simulink subsystem "PvtSubSys_LONC"  (R2020b)
settings: Solver=VariableStepAuto  StartTime=0.0  StopTime=10.0  RelTol=1e-3
undefined symbols (not defined in the file): P_Global_TireRadius_m, P_Global_Weight_N, P_LongCtrl_VLC_fRollCoef, P_LongCtrl_VLC_WindArea, P_LongCtrl_VLCaccelMinHoldXAxis, P_LongCtrl_VLCaccelMinHoldYAxis, P_LongCtrl_VLCaXCDeadZoneProp_Y, P_LongCtrl_VLCaXCKiCtrlDevChar_Y, P_LongCtrl_VLCaxCtrlDevDeadZoneChar_Y, P_LongCtrl_VLCaxCtrlDevEC2DCMax, P_LongCtrl_VLCaxCtrlDevFastQuitDCMode, P_LongCtrl_VLCaxCtrlDevThresAddEC2DC, P_LongCtrl_VLCaxCtrlDevTresAddDC2EC, P_LongCtrl_VLCAxTarDtThreEnableI, P_LongCtrl_VLCaxvRoadSlopeDC4CharXAxis, P_LongCtrl_VLCaxvRoadSlopeDC4CharYAxis, P_LongCtrl_VLCAxvTracMinDC1FullFillXAxis, P_LongCtrl_VLCAxvTracMinDC1FullFillYAxis, P_LongCtrl_VLCcoefFXAxis, P_LongCtrl_VLCcoefFYAxis, P_LongCtrl_VLCcoefIFadeOut1Calc, P_LongCtrl_VLCcoefIFadeOut1Condition, P_LongCtrl_VLCcoefIFadeOut2Calc, P_LongCtrl_VLCcoefIFadeOut2Condition, P_LongCtrl_VLCcoefIFadeOut3Calc, P_LongCtrl_VLCcoefIFadeOut3Condition, P_LongCtrl_VLCCounterAxvTracMinTimeout, P_LongCtrl_VLCCounterDC2ECTorqDelay, P_LongCtrl_VLCCounterDrvOff2EC, P_LongCtrl_VLCdaxTarEC2DCMax, P_LongCtrl_VLCdriveOffAxUpLimXAxix, P_LongCtrl_VLCdriveOffAxUpLimYAxix, P_LongCtrl_VLCDtAxvRef2UpperBandDC5, P_LongCtrl_VLCIACompensionNeg, P_LongCtrl_VLCIACompensionPos, P_LongCtrl_VLCjerkHoldXAxis, P_LongCtrl_VLCjerkHoldYAxis, P_LongCtrl_VLCki, P_LongCtrl_VLCkp, P_LongCtrl_VLCks, P_LongCtrl_VLCTorqDiffThreAxvTracMinTimeout, P_LongCtrl_VLCTrTatioMax, P_LongCtrl_VLCTrTatioMin, P_LongCtrl_VLCVlcAccThresAxvTracMinTimeout
libraries: simulink x32
(part 2 of 2)

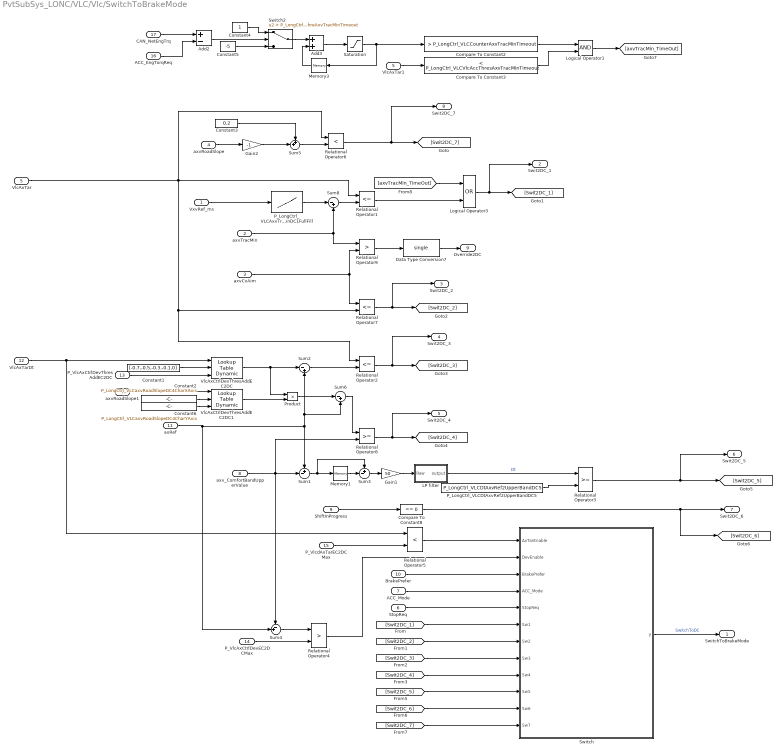
== system PvtSubSys_LONC/VLC/Vlc/SwitchToBrakeMode ==
  VxvRef_ms : Inport
  axvTracMin : Inport  Port=2
  axvCvAim : Inport  Port=3
  axvRoadSlope : Inport  Port=4
  VlcAxTar : Inport  Port=5
  StopReq : Inport  Port=6
  ACC_Mode : Inport  Port=7  OutDataTypeStr=uint8
  axv_ComfortBandUpperValue : Inport  Port=8
  "ShiftInProgress " : Inport  Port=9
  BrakePrefer : Inport  Port=10
  axRef : Inport  Port=11
  VlcAxTarDt : Inport  Port=12
  P_VlcAxCtrlDevThresAddEC2DC : Inport  Port=13
  P_VlcAxCtrlDevEC2DCMax : Inport  Port=14
  P_VlcdAxTarEC2DCMax : Inport  Port=15
  ACC_EngTorqReq : Inport  Port=16  OutDataTypeStr=single
  CAN_NetEngTrq : Inport  Port=17  OutDataTypeStr=single
  Add2 : Sum  Inputs=+-
  Add3 : Sum  AccumDataTypeStr=single
  Compare To Constant2 : simulink/Logic and Bit Operations/Compare To Constant  relop=>  const=P_LongCtrl_VLCCounterAxvTracMinTimeout  OutDataTypeStr=boolean
  Compare To Constant3 : simulink/Logic and Bit Operations/Compare To Constant  relop=<  const=P_LongCtrl_VLCVlcAccThresAxvTracMinTimeout  OutDataTypeStr=boolean
  Compare To Constant8 : simulink/Logic and Bit Operations/Compare To Constant  relop===  const=0  OutDataTypeStr=boolean
  Constant1 : Constant  Value=[-0.7,-0.5,-0.3,-0.1,0]  OutDataTypeStr=single
  Constant2 : Constant  Value=P_LongCtrl_VLCaxvRoadSlopeDC4CharXAxis  OutDataTypeStr=single
  Constant3 : Constant  Value=0.2  OutDataTypeStr=single
  Constant4 : Constant  OutDataTypeStr=single
  Constant5 : Constant  Value=-5  OutDataTypeStr=single
  Constant6 : Constant  Value=P_LongCtrl_VLCaxvRoadSlopeDC4CharYAxis  OutDataTypeStr=single
  Data Type Conversion7 : DataTypeConversion  OutDataTypeStr=single
  Gain1 : Gain  Gain=50
  Gain2 : Gain  Gain=-1
  LP filter : Subsystem
  Logical Operator1 : Logic  AllPortsSameDT=off  OutDataTypeStr=boolean
  Logical Operator3 : Logic  Operator=OR  AllPortsSameDT=off  OutDataTypeStr=boolean
  Memory1 : Memory  InheritSampleTime=on
  Memory3 : Memory  InheritSampleTime=on
  P_LongCtrl_VLCAxvTracMinDC1FullFill : Lookup_n-D  NumberOfTableDimensions=1  BreakpointsForDimension1=P_LongCtrl_VLCAxvTracMinDC1FullFillXAxis  Table=P_LongCtrl_VLCAxvTracMinDC1FullFillYAxis  RndMeth=Simplest  InputSameDT=on
  P_LongCtrl_VLCDtAxvRef2UpperBandDC5 : Constant  Value=P_LongCtrl_VLCDtAxvRef2UpperBandDC5  OutDataTypeStr=single
  Product : Product
  Relational Operator1 : RelationalOperator  Operator=<=  OutDataTypeStr=boolean  RndMeth=Nearest
  Relational Operator2 : RelationalOperator  Operator=<=  OutDataTypeStr=boolean  RndMeth=Nearest
  Relational Operator3 : RelationalOperator  OutDataTypeStr=boolean  RndMeth=Nearest
  Relational Operator4 : RelationalOperator  Operator=>  OutDataTypeStr=boolean  RndMeth=Nearest
  Relational Operator5 : RelationalOperator  Operator=<  OutDataTypeStr=boolean  RndMeth=Nearest
  Relational Operator6 : RelationalOperator  Operator=<  OutDataTypeStr=boolean  RndMeth=Nearest
  Relational Operator7 : RelationalOperator  Operator=<=  OutDataTypeStr=boolean  RndMeth=Nearest
  Relational Operator8 : RelationalOperator  OutDataTypeStr=boolean  RndMeth=Nearest
  Relational Operator9 : RelationalOperator  Operator=>  OutDataTypeStr=boolean  RndMeth=Nearest
  Saturation : Saturate  UpperLimit=100  LowerLimit=0  OutDataTypeStr=single
  Sum1 : Sum  Inputs=+-|
  Sum2 : Sum  Inputs=|-+
  Sum3 : Sum  Inputs=+-|
  Sum4 : Sum  Inputs=-+|
  Sum5 : Sum  Inputs=++|
  Sum6 : Sum  Inputs=|-+
  Sum8 : Sum  Inputs=|-+
  Switch : MATLAB Function  TreatAsAtomicUnit=on
  Switch2 : Switch  Criteria=u2 > Threshold  Threshold=P_LongCtrl_VLCTorqDiffThreAxvTracMinTimeout
  VlcAxCtrlDevThresAddEC2DC : simulink/Lookup Tables/Lookup Table Dynamic  LookUpMeth=Interpolation-Use End Values  OutDataType=fixdt('single')  OutScaling=[]  OutputDataTypeScalingMode=Specify via dialog  OutDataTypeStr=single  DoSatur=off
  VlcAxCtrlDevThresAddEC2DC1 : simulink/Lookup Tables/Lookup Table Dynamic  LookUpMeth=Interpolation-Use End Values  OutDataType=fixdt('single')  OutScaling=[]  OutputDataTypeScalingMode=Specify via dialog  OutDataTypeStr=single  DoSatur=off
  VlcAxTar1 : InportShadow  Port=5
  axvRoadSlope1 : InportShadow  Port=4
  SwitchToBrakeMode : Outport
  Swit2DC_1 : Outport  Port=2
  Swit2DC_2 : Outport  Port=3
  Swit2DC_3 : Outport  Port=4
  Swit2DC_4 : Outport  Port=5
  Swit2DC_5 : Outport  Port=6
  Swit2DC_6 : Outport  Port=7
  Swit2DC_7 : Outport  Port=8
  Override2DC : Outport  Port=9
  wires:
  Product/1 -> Sum6/1
  Constant6/1 -> VlcAxCtrlDevThresAddEC2DC1/3
  axvRoadSlope1/1 -> VlcAxCtrlDevThresAddEC2DC1/1
  VlcAxCtrlDevThresAddEC2DC1/1 -> Product/2
  VlcAxCtrlDevThresAddEC2DC/1 -> Product/1, Sum2/1
  Constant2/1 -> VlcAxCtrlDevThresAddEC2DC1/2
  Sum6/1 -> Relational Operator8/1
  Saturation/1 -> Memory3/1, Compare To Constant2/1
  Relational Operator1/1 -> Logical Operator3/2
  [axvTracMin_TimeOut] -> Logical Operator3/1
  Logical Operator1/1 -> [axvTracMin_TimeOut]
  VlcAxTar1/1 -> Compare To Constant3/1
  ACC_EngTorqReq/1 -> Add2/2
  CAN_NetEngTrq/1 -> Add2/1
  Switch2/1 -> Add3/1
  Constant5/1 -> Switch2/3
  Add2/1 -> Switch2/2
  Compare To Constant3/1 -> Logical Operator1/2
  Compare To Constant2/1 -> Logical Operator1/1
  Add3/1 -> Saturation/1
  Memory3/1 -> Add3/2
  Constant4/1 -> Switch2/1
  Data Type Conversion7/1 -> Override2DC/1
  Relational Operator9/1 -> Data Type Conversion7/1
  axvCvAim/1 -> Relational Operator9/2, Relational Operator7/1
  [Swit2DC_1] -> Switch/6(Sw1)
  [Swit2DC_2] -> Switch/7(Sw2)
  [Swit2DC_3] -> Switch/8(Sw3)
  [Swit2DC_4] -> Switch/9(Sw4)
  [Swit2DC_5] -> Switch/10(Sw5)
  [Swit2DC_6] -> Switch/11(Sw6)
  [Swit2DC_7] -> Switch/12(Sw7)
  StopReq/1 -> Switch/5(StopReq)
  ACC_Mode/1 -> Switch/4(ACC_Mode)
  BrakePrefer/1 -> Switch/3(BrakePrefer)
  Relational Operator4/1 -> Switch/2(DevEnable)
  Relational Operator5/1 -> Switch/1(AxTarEnable)
  Compare To Constant8/1 -> Swit2DC_6/1, [Swit2DC_6]
  "ShiftInProgress "/1 -> Compare To Constant8/1
  Relational Operator3/1 -> Swit2DC_5/1, [Swit2DC_5]
  Relational Operator8/1 -> Swit2DC_4/1, [Swit2DC_4]
  Relational Operator2/1 -> Swit2DC_3/1, [Swit2DC_3]
  Relational Operator7/1 -> [Swit2DC_2], Swit2DC_2/1
  Logical Operator3/1 -> [Swit2DC_1], Swit2DC_1/1
  Relational Operator6/1 -> [Swit2DC_7], Swit2DC_7/1
  Sum5/1 -> Relational Operator6/2
  VlcAxTar/1 -> Relational Operator6/1, Relational Operator1/1, Relational Operator2/1, Relational Operator7/2
  Constant3/1 -> Sum5/1
  Gain2/1 -> Sum5/2
  axvRoadSlope/1 -> Gain2/1
  P_LongCtrl_VLCAxvTracMinDC1FullFill/1 -> Sum8/1
  P_VlcdAxTarEC2DCMax/1 -> Relational Operator5/2
  P_VlcAxCtrlDevEC2DCMax/1 -> Relational Operator4/2
  Sum4/1 -> Relational Operator4/1
  axv_ComfortBandUpperValue/1 -> Sum4/1, Sum1/2, Relational Operator8/2
  P_LongCtrl_VLCDtAxvRef2UpperBandDC5/1 -> Relational Operator3/2
  P_VlcAxCtrlDevThresAddEC2DC/1 -> VlcAxCtrlDevThresAddEC2DC/3
  Constant1/1 -> VlcAxCtrlDevThresAddEC2DC/2
  VlcAxTarDt/1 -> Relational Operator5/1, VlcAxCtrlDevThresAddEC2DC/1
  LP filter/1(output) -> Relational Operator3/1  "Dt"
  Gain1/1 -> LP filter/1(Raw)
  Sum3/1 -> Gain1/1
  Memory1/1 -> Sum3/2
  Sum2/1 -> Relational Operator2/2
  Sum1/1 -> Sum3/1, Memory1/1
  axRef/1 -> Sum1/1, Sum6/2, Sum2/2, Sum4/2
  Switch/1(y) -> SwitchToBrakeMode/1  "SwitchToDC"
  Sum8/1 -> Relational Operator1/2
  axvTracMin/1 -> Sum8/2, Relational Operator9/1
  VxvRef_ms/1 -> P_LongCtrl_VLCAxvTracMinDC1FullFill/1

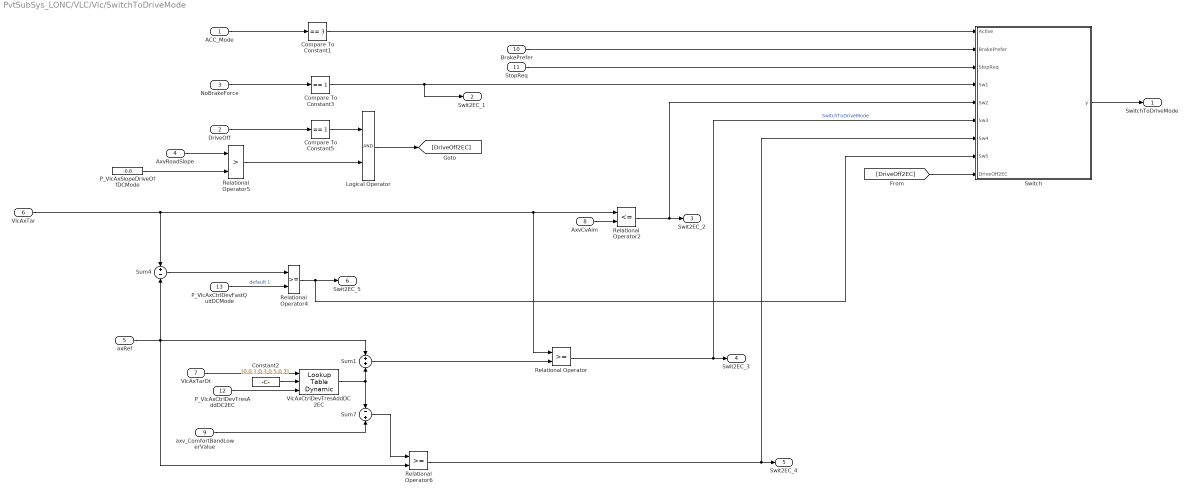
== system PvtSubSys_LONC/VLC/Vlc/SwitchToDriveMode ==
  ACC_Mode : Inport
  DriveOff : Inport  Port=2
  NoBrakeForce : Inport  Port=3
  AxvRoadSlope : Inport  Port=4
  axRef : Inport  Port=5
  VlcAxTar : Inport  Port=6
  VlcAxTarDt : Inport  Port=7
  AxvCvAim : Inport  Port=8
  axv_ComfortBandLowerValue : Inport  Port=9
  BrakePrefer : Inport  Port=10
  StopReq : Inport  Port=11
  P_VlcAxCtrlDevTresAddDC2EC : Inport  Port=12
  P_VlcAxCtrlDevFastQuitDCMode : Inport  Port=13
  Compare To Constant1 : simulink/Logic and Bit Operations/Compare To Constant  relop===  const=3  OutDataTypeStr=boolean
  Compare To Constant3 : simulink/Logic and Bit Operations/Compare To Constant  relop===  const=1  OutDataTypeStr=boolean
  Compare To Constant5 : simulink/Logic and Bit Operations/Compare To Constant  relop===  const=1  OutDataTypeStr=boolean
  Constant2 : Constant  Value=[0,0.1,0.3,0.5,0.7]  OutDataTypeStr=single
  Logical Operator : Logic  AllPortsSameDT=off  OutDataTypeStr=boolean
  P_VlcAxSlopeDriveOffDCMode : Constant  Value=-0.8
  Relational Operator : RelationalOperator  OutDataTypeStr=boolean  RndMeth=Nearest
  Relational Operator2 : RelationalOperator  Operator=<=  OutDataTypeStr=boolean  RndMeth=Nearest
  Relational Operator4 : RelationalOperator  OutDataTypeStr=boolean  RndMeth=Nearest
  Relational Operator5 : RelationalOperator  Operator=>  OutDataTypeStr=boolean  RndMeth=Nearest
  Relational Operator6 : RelationalOperator  OutDataTypeStr=boolean  RndMeth=Nearest
  Sum1 : Sum
  Sum4 : Sum  Inputs=+-
  Sum7 : Sum  Inputs=-+
  Switch : MATLAB Function  TreatAsAtomicUnit=on
  VlcAxCtrlDevTresAddDC2EC : simulink/Lookup Tables/Lookup Table Dynamic  LookUpMeth=Interpolation-Use End Values  OutDataType=fixdt('double')  OutScaling=[]  OutputDataTypeScalingMode=Specify via dialog  OutDataTypeStr=fixdt('double')  DoSatur=off
  SwitchToDriveMode : Outport
  Swit2EC_1 : Outport  Port=2
  Swit2EC_2 : Outport  Port=3
  Swit2EC_3 : Outport  Port=4
  Swit2EC_4 : Outport  Port=5
  Swit2EC_5 : Outport  Port=6
  wires:
  StopReq/1 -> Switch/3(StopReq)
  [DriveOff2EC] -> Switch/9(DriveOff2EC)
  Compare To Constant3/1 -> Switch/4(Sw1), Swit2EC_1/1
  Relational Operator2/1 -> Swit2EC_2/1, Switch/5(Sw2)
  Relational Operator6/1 -> Swit2EC_4/1, Switch/7(Sw4)
  Relational Operator4/1 -> Swit2EC_5/1, Switch/8(Sw5)
  BrakePrefer/1 -> Switch/2(BrakePrefer)
  Sum4/1 -> Relational Operator4/1
  axv_ComfortBandLowerValue/1 -> Sum7/2
  Relational Operator/1 -> Swit2EC_3/1, Switch/6(Sw3)  "SwitchToDriveMode"
  Sum7/1 -> Relational Operator6/1
  Sum1/1 -> Relational Operator/2
  AxvCvAim/1 -> Relational Operator2/2
  VlcAxTar/1 -> Sum4/1, Relational Operator2/1, Relational Operator/1
  Relational Operator5/1 -> Logical Operator/2
  P_VlcAxSlopeDriveOffDCMode/1 -> Relational Operator5/2
  AxvRoadSlope/1 -> Relational Operator5/1
  Switch/1(y) -> SwitchToDriveMode/1
  P_VlcAxCtrlDevFastQuitDCMode/1 -> Relational Operator4/2  "default 1"
  axRef/1 -> Relational Operator6/2, Sum1/1, Sum4/2
  Compare To Constant1/1 -> Switch/1(Active)
  Logical Operator/1 -> [DriveOff2EC]
  Compare To Constant5/1 -> Logical Operator/1
  DriveOff/1 -> Compare To Constant5/1
  ACC_Mode/1 -> Compare To Constant1/1
  VlcAxCtrlDevTresAddDC2EC/1 -> Sum7/1, Sum1/2
  P_VlcAxCtrlDevTresAddDC2EC/1 -> VlcAxCtrlDevTresAddDC2EC/3
  Constant2/1 -> VlcAxCtrlDevTresAddDC2EC/2
  VlcAxTarDt/1 -> VlcAxCtrlDevTresAddDC2EC/1
  NoBrakeForce/1 -> Compare To Constant3/1

== system PvtSubSys_LONC/VLC/Vlc/UpdateFlagCalc ==
  NoBrakeForce : Inport
  DCT_ShiftInProgress : Inport  Port=2
  AxRefDt : Inport  Port=3
  Vxv : Inport  Port=4
  Abs4 : Abs
  Compare To Constant1 : simulink/Logic and Bit Operations/Compare To Constant  relop=<=  const=5  OutDataTypeStr=boolean
  Compare To Constant2 : simulink/Logic and Bit Operations/Compare To Constant  relop=>=  const=18  OutDataTypeStr=boolean
  Compare To Constant4 : simulink/Logic and Bit Operations/Compare To Constant  relop===  const=0  OutDataTypeStr=boolean
  Compare To Constant7 : simulink/Logic and Bit Operations/Compare To Constant  relop===  const=6  OutDataTypeStr=boolean
  Compare To Constant8 : simulink/Logic and Bit Operations/Compare To Constant  relop===  const=0  OutDataTypeStr=boolean
  Logical Operator : Logic  Inputs=5  AllPortsSameDT=off  OutDataTypeStr=boolean
  Sum of Elements1 : Sum  Inputs=+
  Tapped Delay1 : simulink/Discrete/Tapped Delay  vinit=0.0  samptime=-1  NumDelays=5  DelayOrder=Newest  includeCurrent=on
  Timer : Subsystem
  UpdateEnable : Outport
  wires:
  Vxv/1 -> Compare To Constant2/1
  Compare To Constant1/1 -> Logical Operator/2
  Logical Operator/1 -> UpdateEnable/1
  NoBrakeForce/1 -> Tapped Delay1/1
  Timer/1(Timer) -> Compare To Constant4/1
  Compare To Constant7/1 -> Logical Operator/1
  Compare To Constant4/1 -> Logical Operator/5
  DCT_ShiftInProgress/1 -> Compare To Constant8/1, Timer/1(Falling)
  AxRefDt/1 -> Abs4/1
  Tapped Delay1/1 -> Sum of Elements1/1
  Sum of Elements1/1 -> Compare To Constant7/1
  Compare To Constant2/1 -> Logical Operator/3
  Compare To Constant8/1 -> Logical Operator/4
  Abs4/1 -> Compare To Constant1/1

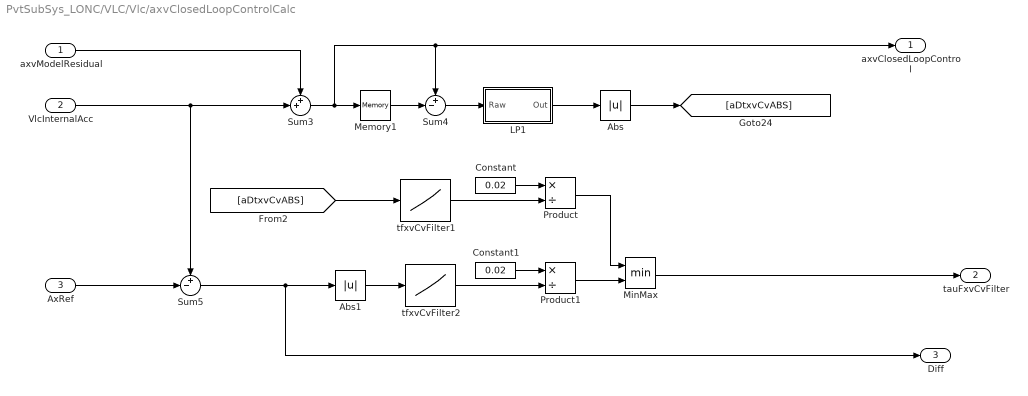
== system PvtSubSys_LONC/VLC/Vlc/axvClosedLoopControlCalc ==
  axvModelResidual : Inport
  VlcInternalAcc : Inport  Port=2
  AxRef : Inport  Port=3
  Abs : Abs
  Abs1 : Abs
  Constant : Constant  Value=0.02  OutDataTypeStr=single
  Constant1 : Constant  Value=0.02  OutDataTypeStr=single
  LP1 : Subsystem
  Memory1 : Memory  InheritSampleTime=on
  MinMax : MinMax  Inputs=2
  Product : Product  Inputs=*/  RndMeth=Zero
  Product1 : Product  Inputs=*/  RndMeth=Zero
  Sum3 : Sum  Inputs=++|
  Sum4 : Sum  Inputs=+-|
  Sum5 : Sum  Inputs=+-|
  "tfxvCvFilter1 " : Lookup_n-D  NumberOfTableDimensions=1  BreakpointsForDimension1=[0,0.1,0.2,1]  Table=[0.1,0.1,0.04,0.04]  RndMeth=Simplest  InputSameDT=on
  tfxvCvFilter2 : Lookup_n-D  NumberOfTableDimensions=1  BreakpointsForDimension1=[0,0.1,0.2,1]  Table=[0.1,0.1,0.02,0.02]  RndMeth=Simplest  InputSameDT=on
  axvClosedLoopControl : Outport
  tauFxvCvFilter : Outport  Port=2
  Diff : Outport  Port=3
  wires:
  AxRef/1 -> Sum5/2
  LP1/1(Out) -> Abs/1
  axvModelResidual/1 -> Sum3/1
  MinMax/1 -> tauFxvCvFilter/1
  Product1/1 -> MinMax/2
  Product/1 -> MinMax/1
  tfxvCvFilter2/1 -> Product1/2
  Constant1/1 -> Product1/1
  "tfxvCvFilter1 "/1 -> Product/2
  Constant/1 -> Product/1
  Abs1/1 -> tfxvCvFilter2/1
  Sum5/1 -> Abs1/1, Diff/1
  VlcInternalAcc/1 -> Sum3/2, Sum5/1
  [aDtxvCvABS] -> "tfxvCvFilter1 "/1
  Abs/1 -> [aDtxvCvABS]
  Sum4/1 -> LP1/1(Raw)
  Memory1/1 -> Sum4/2
  Sum3/1 -> Memory1/1, Sum4/1, axvClosedLoopControl/1

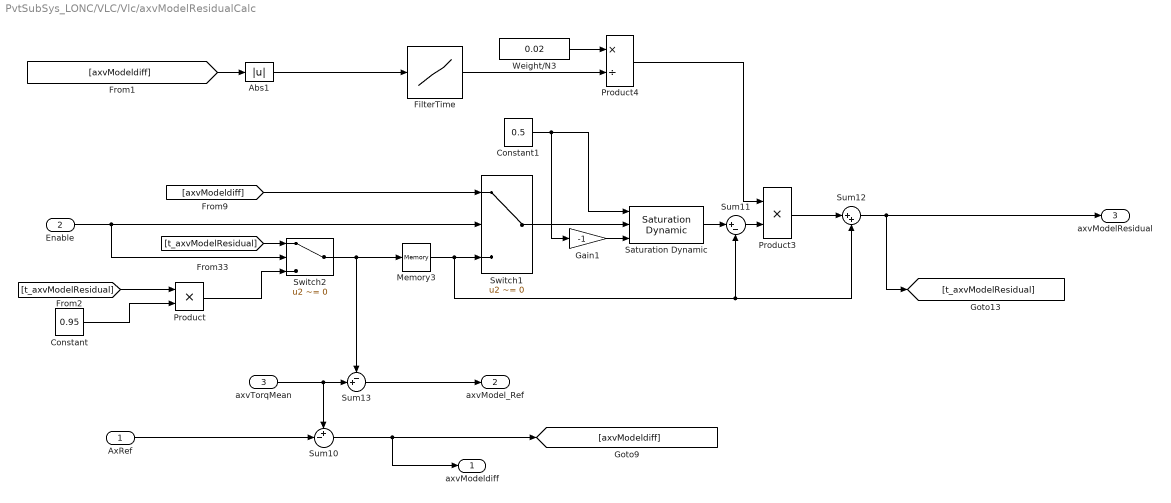
== system PvtSubSys_LONC/VLC/Vlc/axvModelResidualCalc ==
  AxRef : Inport
  Enable : Inport  Port=2
  axvTorqMean : Inport  Port=3
  Abs1 : Abs
  Constant : Constant  Value=0.95  OutDataTypeStr=single
  Constant1 : Constant  Value=0.5  OutDataTypeStr=single
  FilterTime : Lookup_n-D  NumberOfTableDimensions=1  BreakpointsForDimension1=[0,0.1,0.4,0.8,1]  Table=[1,0.4,0.1,0.04,0.04]  RndMeth=Simplest  InputSameDT=on
  Gain1 : Gain  Gain=-1
  Memory3 : Memory  InheritSampleTime=on
  Product : Product  OutDataTypeStr=single
  Product3 : Product  RndMeth=Zero
  Product4 : Product  Inputs=*/  RndMeth=Zero
  Saturation Dynamic : simulink/Discontinuities/Saturation Dynamic  OutMin=[]  OutMax=[]  OutDataTypeStr=Inherit: Same as second input  OutDataType=fixdt(1, 16)  OutScaling=2^-10  DoSatur=off
  Sum10 : Sum  Inputs=+-|
  Sum11 : Sum  Inputs=|+-
  Sum12 : Sum  Inputs=|++
  Sum13 : Sum  Inputs=-+|
  Switch1 : Switch  Criteria=u2 ~= 0
  Switch2 : Switch  Criteria=u2 ~= 0  OutDataTypeStr=single
  Weight/N3 : Constant  Value=0.02  OutDataTypeStr=single  SampleTime=-1
  axvModeldiff : Outport
  axvModel_Ref : Outport  Port=2
  axvModelResidual : Outport  Port=3
  wires:
  Sum13/1 -> axvModel_Ref/1
  Constant/1 -> Product/2
  Constant1/1 -> Saturation Dynamic/1, Gain1/1
  axvTorqMean/1 -> Sum13/2, Sum10/1
  [t_axvModelResidual] -> Switch2/1
  Product3/1 -> Sum12/1
  Saturation Dynamic/1 -> Sum11/1
  [t_axvModelResidual] -> Product/1
  Enable/1 -> Switch1/2, Switch2/2
  Gain1/1 -> Saturation Dynamic/3
  AxRef/1 -> Sum10/2
  [axvModeldiff] -> Abs1/1
  Abs1/1 -> FilterTime/1
  Sum12/1 -> [t_axvModelResidual], axvModelResidual/1
  Sum10/1 -> axvModeldiff/1, [axvModeldiff]
  FilterTime/1 -> Product4/2
  [axvModeldiff] -> Switch1/1
  Switch2/1 -> Memory3/1, Sum13/1
  Product/1 -> Switch2/3
  Memory3/1 -> Switch1/3, Sum11/2, Sum12/2
  Product4/1 -> Product3/1
  Switch1/1 -> Saturation Dynamic/2
  Weight/N3/1 -> Product4/1
  Sum11/1 -> Product3/2

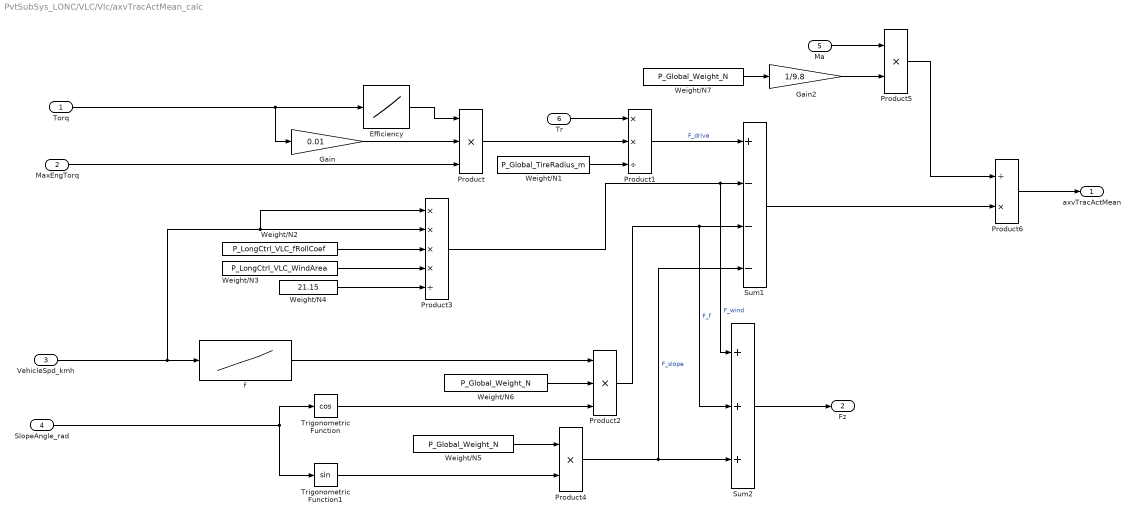
== system PvtSubSys_LONC/VLC/Vlc/axvTracActMean_calc ==
  Torq : Inport  OutDataTypeStr=single
  MaxEngTorq : Inport  Port=2  OutDataTypeStr=single
  VehicleSpd_kmh : Inport  Port=3  OutDataTypeStr=single
  SlopeAngle_rad : Inport  Port=4  OutDataTypeStr=single
  Ma : Inport  Port=5  OutDataTypeStr=single
  Tr : Inport  Port=6  OutDataTypeStr=single
  Efficiency : Lookup_n-D  NumberOfTableDimensions=1  BreakpointsForDimension1=[-100,-20,0,20,100]  Table=[1.10,1.10,1,0.90,0.90]  RndMeth=Simplest  InputSameDT=on
  Gain : Gain  Gain=0.01
  Gain2 : Gain  Gain=1/9.8
  Product : Product  Inputs=***  RndMeth=Zero
  Product1 : Product  Inputs=**/  RndMeth=Zero
  Product2 : Product  Inputs=***  RndMeth=Zero
  Product3 : Product  Inputs=****/  RndMeth=Zero
  Product4 : Product  Inputs=**  RndMeth=Zero
  Product5 : Product  Inputs=**  RndMeth=Zero
  Product6 : Product  Inputs=/*  RndMeth=Zero
  Sum1 : Sum  Inputs=+---
  Sum2 : Sum  Inputs=+++
  Trigonometric Function : Trigonometry  Operator=cos
  Trigonometric Function1 : Trigonometry
  Weight/N1 : Constant  Value=P_Global_TireRadius_m  OutDataTypeStr=single
  Weight/N2 : Constant  Value=P_LongCtrl_VLC_fRollCoef  OutDataTypeStr=single
  Weight/N3 : Constant  Value=P_LongCtrl_VLC_WindArea  OutDataTypeStr=single
  Weight/N4 : Constant  Value=21.15  OutDataTypeStr=single
  Weight/N5 : Constant  Value=P_Global_Weight_N  OutDataTypeStr=single
  Weight/N6 : Constant  Value=P_Global_Weight_N  OutDataTypeStr=single
  Weight/N7 : Constant  Value=P_Global_Weight_N  OutDataTypeStr=single
  f : Lookup_n-D  NumberOfTableDimensions=1  BreakpointsForDimension1=P_LongCtrl_VLCcoefFXAxis  Table=P_LongCtrl_VLCcoefFYAxis  RndMeth=Simplest  InputSameDT=on
  axvTracActMean : Outport  OutDataTypeStr=single
  Fz : Outport  Port=2  OutDataTypeStr=single
  wires:
  f/1 -> Product2/1
  Weight/N1/1 -> Product1/3
  Weight/N5/1 -> Product4/1
  Weight/N6/1 -> Product2/2
  Weight/N7/1 -> Gain2/1
  Sum2/1 -> Fz/1
  Trigonometric Function1/1 -> Product4/2
  Product6/1 -> axvTracActMean/1
  MaxEngTorq/1 -> Product/3
  Tr/1 -> Product1/1
  Ma/1 -> Product5/1
  Gain2/1 -> Product5/2
  Product5/1 -> Product6/1
  Sum1/1 -> Product6/2
  Product4/1 -> Sum1/4, Sum2/3  "F_slope"
  Product2/1 -> Sum1/3, Sum2/2  "F_f"
  Product3/1 -> Sum1/2, Sum2/1  "F_wind"
  Weight/N4/1 -> Product3/5
  Weight/N3/1 -> Product3/4
  Weight/N2/1 -> Product3/3
  Product1/1 -> Sum1/1  "F_drive"
  Trigonometric Function/1 -> Product2/3
  SlopeAngle_rad/1 -> Trigonometric Function1/1, Trigonometric Function/1
  VehicleSpd_kmh/1 -> Product3/1, Product3/2, f/1
  Product/1 -> Product1/2
  Gain/1 -> Product/2
  Efficiency/1 -> Product/1
  Torq/1 -> Efficiency/1, Gain/1

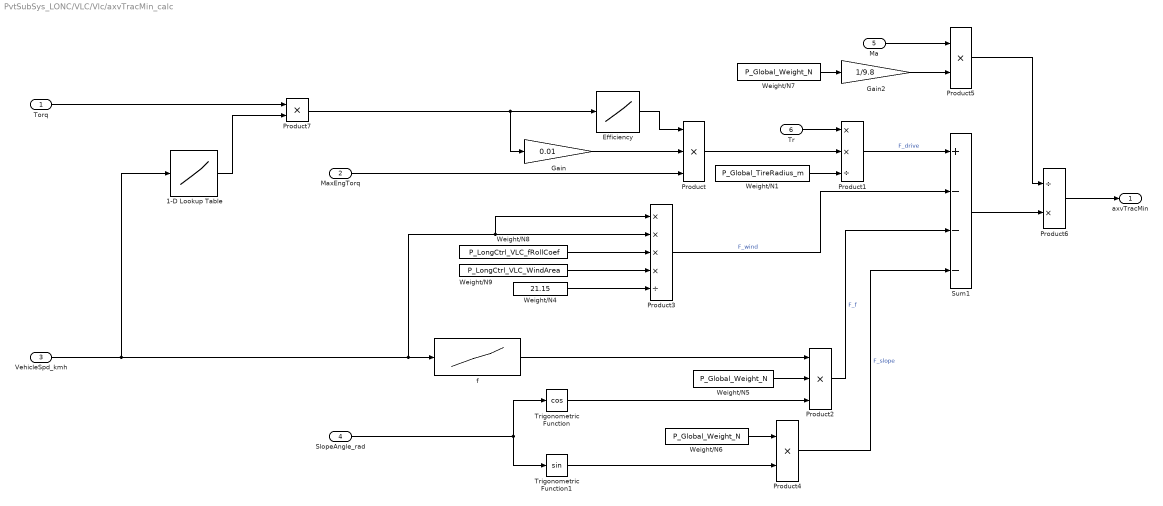
== system PvtSubSys_LONC/VLC/Vlc/axvTracMin_calc ==
  Torq : Inport
  MaxEngTorq : Inport  Port=2
  VehicleSpd_kmh : Inport  Port=3
  SlopeAngle_rad : Inport  Port=4
  Ma : Inport  Port=5
  Tr : Inport  Port=6
  1-D Lookup Table : Lookup_n-D  NumberOfTableDimensions=1  BreakpointsForDimension1=[0 10 20 30 40 50 60 70 80 90 100]  Table=[0 0 0.1 0.65 0.75 0.8 0.85 0.9 0.95 1 1]  ExtrapMethod=Clip  InternalRulePriority=Speed  RndMeth=Simplest  InputSameDT=on
  Efficiency : Lookup_n-D  NumberOfTableDimensions=1  BreakpointsForDimension1=[-100,-20,0,20,100]  Table=[1.10,1.10,1,0.90,0.90]  RndMeth=Simplest  InputSameDT=on
  Gain : Gain  Gain=0.01
  Gain2 : Gain  Gain=1/9.8
  Product : Product  Inputs=***  RndMeth=Zero
  Product1 : Product  Inputs=**/  RndMeth=Zero
  Product2 : Product  Inputs=***  RndMeth=Zero
  Product3 : Product  Inputs=****/  RndMeth=Zero
  Product4 : Product  Inputs=**  RndMeth=Zero
  Product5 : Product  Inputs=**  RndMeth=Zero
  Product6 : Product  Inputs=/*  RndMeth=Zero
  Product7 : Product
  Sum1 : Sum  Inputs=+---
  Trigonometric Function : Trigonometry  Operator=cos
  Trigonometric Function1 : Trigonometry
  Weight/N1 : Constant  Value=P_Global_TireRadius_m  OutDataTypeStr=single
  Weight/N4 : Constant  Value=21.15  OutDataTypeStr=single
  Weight/N5 : Constant  Value=P_Global_Weight_N  OutDataTypeStr=single
  Weight/N6 : Constant  Value=P_Global_Weight_N  OutDataTypeStr=single
  Weight/N7 : Constant  Value=P_Global_Weight_N  OutDataTypeStr=single
  Weight/N8 : Constant  Value=P_LongCtrl_VLC_fRollCoef  OutDataTypeStr=single
  Weight/N9 : Constant  Value=P_LongCtrl_VLC_WindArea  OutDataTypeStr=single
  f : Lookup_n-D  NumberOfTableDimensions=1  BreakpointsForDimension1=P_LongCtrl_VLCcoefFXAxis  Table=P_LongCtrl_VLCcoefFYAxis  RndMeth=Simplest  InputSameDT=on
  axvTracMin : Outport
  wires:
  Torq/1 -> Product7/1
  1-D Lookup Table/1 -> Product7/2
  Product7/1 -> Efficiency/1, Gain/1
  Tr/1 -> Product1/1
  Ma/1 -> Product5/1
  f/1 -> Product2/1
  Weight/N1/1 -> Product1/3
  Weight/N6/1 -> Product4/1
  Weight/N5/1 -> Product2/2
  Weight/N7/1 -> Gain2/1
  Trigonometric Function1/1 -> Product4/2
  Product6/1 -> axvTracMin/1
  MaxEngTorq/1 -> Product/3
  Gain2/1 -> Product5/2
  Product5/1 -> Product6/1
  Sum1/1 -> Product6/2
  Product4/1 -> Sum1/4  "F_slope"
  Product2/1 -> Sum1/3  "F_f"
  Product3/1 -> Sum1/2  "F_wind"
  Weight/N4/1 -> Product3/5
  Weight/N9/1 -> Product3/4
  Weight/N8/1 -> Product3/3
  Product1/1 -> Sum1/1  "F_drive"
  Trigonometric Function/1 -> Product2/3
  SlopeAngle_rad/1 -> Trigonometric Function1/1, Trigonometric Function/1
  VehicleSpd_kmh/1 -> Product3/1, Product3/2, f/1, 1-D Lookup Table/1
  Product/1 -> Product1/2
  Gain/1 -> Product/2
  Efficiency/1 -> Product/1

== system PvtSubSys_LONC/VLC/Vlc/EC/LP ==
  Raw : Inport
  Constant1 : Constant  Value=0.05  OutDataTypeStr=single
  Constant3 : Constant  Value=0.02  OutDataTypeStr=single
  Memory8 : Memory  InheritSampleTime=on
  Product7 : Product  Inputs=*/  RndMeth=Zero
  Product8 : Product  RndMeth=Zero
  Sum14 : Sum
  Sum9 : Sum  Inputs=|+-
  Out : Outport
  wires:
  Constant1/1 -> Product7/2
  Constant3/1 -> Product7/1
  Sum9/1 -> Product8/2
  Sum14/1 -> Memory8/1, Out/1
  Memory8/1 -> Sum14/2, Sum9/2
  Raw/1 -> Sum9/1
  Product8/1 -> Sum14/1
  Product7/1 -> Product8/1

== system PvtSubSys_LONC/VLC/Vlc/FF_Control/L  P ==
  Raw : Inport
  VxvRef : Inport  Port=2
  Constant2 : Constant  Value=0.02  OutDataTypeStr=single
  FilterTime : Lookup_n-D  NumberOfTableDimensions=1  BreakpointsForDimension1=[0,10,20,30,40]  Table=[0.5,0.5,2,3,3]  RndMeth=Simplest  InputSameDT=on
  Memory4 : Memory  InheritSampleTime=on
  Product2 : Product  Inputs=*/  RndMeth=Zero
  Product6 : Product  OutDataTypeStr=single  RndMeth=Zero
  Sum6 : Sum  Inputs=+-
  Sum7 : Sum
  Out : Outport
  wires:
  VxvRef/1 -> FilterTime/1
  Raw/1 -> Sum6/1
  Product6/1 -> Sum7/1
  Product2/1 -> Product6/1
  Sum6/1 -> Product6/2
  FilterTime/1 -> Product2/2
  Constant2/1 -> Product2/1
  Memory4/1 -> Sum7/2, Sum6/2
  Sum7/1 -> Memory4/1, Out/1

== system PvtSubSys_LONC/VLC/Vlc/FF_Control/LP ==
  Raw : Inport
  tauFxvCvFilter : Inport  Port=2
  Add2 : Sum  Inputs=+-
  Add3 : Sum
  Memory : Memory  InheritSampleTime=on
  Product4 : Product  Inputs=**  RndMeth=Zero
  Out : Outport
  wires:
  tauFxvCvFilter/1 -> Product4/1
  Product4/1 -> Add3/1
  Add3/1 -> [FxvCv]
  Add2/1 -> Product4/2
  Memory/1 -> Add2/2, Add3/2
  [FxvCv] -> Memory/1, Out/1
  Raw/1 -> Add2/1

== system PvtSubSys_LONC/VLC/Vlc/PI_Control/If Action Subsystem ==
  In1 : Inport
  Action Port : ActionPort
  Out1 : Outport
  wires:
  In1/1 -> Out1/1

== system PvtSubSys_LONC/VLC/Vlc/PI_Control/If Action Subsystem1 ==
  In1 : Inport
  Action Port : ActionPort
  Gain2 : Gain  Gain=-1
  Out1 : Outport
  wires:
  Gain2/1 -> Out1/1
  In1/1 -> Gain2/1

== system PvtSubSys_LONC/VLC/Vlc/SwitchToBrakeMode/LP filter ==
  Raw : Inport
  FilterTime : Constant  Value=0.1  OutDataTypeStr=single
  Memory2 : Memory  InheritSampleTime=on
  Product1 : Product  RndMeth=Zero
  Product4 : Product  Inputs=*/  RndMeth=Zero
  Sum4 : Sum  Inputs=+-|
  Sum5 : Sum  Inputs=++|
  Weight/N3 : Constant  Value=0.02  OutDataTypeStr=single
  output : Outport
  wires:
  Memory2/1 -> Sum4/2, Sum5/2
  Sum4/1 -> Product1/2
  Sum5/1 -> Memory2/1, output/1
  Product1/1 -> Sum5/1
  Raw/1 -> Sum4/1
  Weight/N3/1 -> Product4/1
  Product4/1 -> Product1/1
  FilterTime/1 -> Product4/2

== system PvtSubSys_LONC/VLC/Vlc/UpdateFlagCalc/Timer ==
  Falling : Inport
  Detect Decrease : simulink/Logic and Bit Operations/Detect Decrease  vinit=0.0  OutDataTypeStr=uint8
  MATLAB Function : MATLAB Function  TreatAsAtomicUnit=on
  Unit Delay : UnitDelay  SampleTime=-1  HasFrameUpgradeWarning=on
  Unit Delay1 : UnitDelay  SampleTime=-1  HasFrameUpgradeWarning=on
  Timer : Outport
  wires:
  Unit Delay/1 -> MATLAB Function/3(StartTimerK1)
  Detect Decrease/1 -> MATLAB Function/1(Falling)
  Unit Delay1/1 -> MATLAB Function/2(TimerK1)
  MATLAB Function/2(StartTimer) -> Unit Delay/1
  Falling/1 -> Detect Decrease/1
  MATLAB Function/1(Timer) -> Unit Delay1/1, Timer/1

== system PvtSubSys_LONC/VLC/Vlc/axvClosedLoopControlCalc/LP1 ==
  Raw : Inport
  Constant3 : Constant  Value=0.02  OutDataTypeStr=single
  FilterTime2 : Constant  Value=0.1  OutDataTypeStr=single
  Memory8 : Memory  InheritSampleTime=on
  Product7 : Product  Inputs=*/  RndMeth=Zero
  Product8 : Product  RndMeth=Zero
  Sum14 : Sum
  Sum9 : Sum  Inputs=+-
  Out : Outport
  wires:
  Constant3/1 -> Product7/1
  FilterTime2/1 -> Product7/2
  Sum9/1 -> Product8/2
  Sum14/1 -> Memory8/1, Out/1
  Memory8/1 -> Sum14/2, Sum9/2
  Raw/1 -> Sum9/1
  Product8/1 -> Sum14/1
  Product7/1 -> Product8/1

== stateflow chart PvtSubSys_LONC/VLC/Vlc/DC/StandstillAccel2 ==
  (default) -> (junction 1)
  (junction 1) -> (junction 3) [order 1] : [ACCmode(1)==6||ACCmode(1)==9]
  (junction 1) -> (junction 7) [order 2] : {timer=single(0);
      | decelReq=VlcAxTar;}
  (junction 3) -> (junction 5) : {timer=min(single(100),timer+single(1));
      |  Ax=min(single(-0.3),VlcAxTar);
      | decelReq=max(accelHoldMin,(Ax+jerkHold*single(0.02)*timer));}
  (junction 5) -> (junction 7)
  (junction 7) -> (junction 14)
  (junction 14) -> (junction 19) [order 1] : [(ACCmode(2)==6||ACCmode(2)==9)&&(ACCmode(1)==7)]
  (junction 14) -> (junction 23) [order 2] : {timerFailure=max(uint8(0),timerFailure-uint8(1));}
  (junction 19) -> (junction 21) : {timerFailure=uint8(75);}
  (junction 21) -> (junction 23)
  (junction 23) -> (junction 26)
  (junction 26) -> (junction 28) [order 1] : [timerFailure>0]
  (junction 26) -> (junction 32) [order 2] : {decelReqActive=false;}
  (junction 28) -> (junction 30) : {decelReq=decelReqK1;
      |  decelReqActive=true;}
  (junction 30) -> (junction 32)
  (junction 32) -> (junction 35) : {decelReqK1=decelReq;}
  data: decelReqActive output; VlcAxTar input single; ACCmode input; timer local single =single(0); decelReq output single; Ax local; accelHoldMin input; jerkHold input single; timerFailure local =uint8(0); decelReqK1 local

== matlab function PvtSubSys_LONC/VLC/Vlc/EC/FxLimit ==
  data: tEC input single; Up output single; UpDelta input single; VxvRef input single; LowDelta input single; DCK1 input boolean; EC input boolean; Driveoff input boolean; CounterK1 input single; Low output single; Counter output single; Counter2K1 input single; Counter2 output single; P_LongCtrl_VLCCounterDrvOff2EC parameter single; P_LongCtrl_VLCCounterDC2ECTorqDelay parameter single
function [Up,Low,Counter,Counter2] = fcn(tEC,UpDelta,VxvRef,LowDelta,DCK1,EC,Driveoff,CounterK1,Counter2K1, P_LongCtrl_VLCCounterDrvOff2EC, P_LongCtrl_VLCCounterDC2ECTorqDelay)
%#codegen
Counter = single(max(CounterK1-1,single(0))); 
Counter2 = single(max(Counter2K1-1,single(0))); 
if ((Driveoff(1)==1)&&(Driveoff(2)==0))
    Counter=P_LongCtrl_VLCCounterDrvOff2EC;             
else
    if (VxvRef>0.3)&&(EC(1)==1)&&(DCK1==1)
        Counter2=P_LongCtrl_VLCCounterDC2ECTorqDelay;         
    end
end
if ( Counter>0)
    Up=single(0);
    Low=single(0);
else
    Up = min(tEC*single(0.5),UpDelta);
    Low = max(-tEC, LowDelta);
    if Counter2>0
        Up = min(tEC*single(0.1),UpDelta);
    end
end

== matlab function PvtSubSys_LONC/VLC/Vlc/EC/MATLAB Function ==
  data: EngTorq_k1 input; NetEngTorq input; y output; EC_enable_k1 input
function y = fcn(EngTorq_k1,NetEngTorq,EC_enable_k1)
%#codegen
if EC_enable_k1==0
    y = NetEngTorq;
else
    y = EngTorq_k1;
end

== matlab function PvtSubSys_LONC/VLC/Vlc/PI_Control/MATLAB Function ==
  data: I_k1 input single; Err input single; ECenable input boolean; I output single; Limited output single; axvFilt output single; Diff input single; tCycle input single; P_VlcWindupLim input single; AxTarDt input single; axv input single; tConst input single; VlcAxTar input single; ShiftInProgress input boolean; axvFiltK1 input single; P_LongCtrl_VLCAxTarDtThreEnableI parameter single; P_LongCtrl_VLCcoefIFadeOut1Condition parameter single; P_LongCtrl_VLCcoefIFadeOut1Calc parameter single; P_LongCtrl_VLCcoefIFadeOut2Condition parameter single; P_LongCtrl_VLCcoefIFadeOut2Calc parameter single; P_LongCtrl_VLCcoefIFadeOut3Condition parameter single; P_LongCtrl_VLCcoefIFadeOut3Calc parameter single; P_LongCtrl_VLCIACompensionPos parameter single; P_LongCtrl_VLCIACompensionNeg parameter single
function [I,Limited,axvFilt] = calcI(I_k1,Err,ECenable,Diff,tCycle,P_VlcWindupLim,AxTarDt,axv,tConst,VlcAxTar,ShiftInProgress,axvFiltK1,P_LongCtrl_VLCAxTarDtThreEnableI, P_LongCtrl_VLCcoefIFadeOut1Condition, P_LongCtrl_VLCcoefIFadeOut1Calc, P_LongCtrl_VLCcoefIFadeOut2Condition, P_LongCtrl_VLCcoefIFadeOut2Calc,...
      P_LongCtrl_VLCcoefIFadeOut3Condition, P_LongCtrl_VLCcoefIFadeOut3Calc, P_LongCtrl_VLCIACompensionPos, P_LongCtrl_VLCIACompensionNeg)
tau=tCycle/tConst;
axvFilt=tau*(axv-axvFiltK1)+axvFiltK1;
if ShiftInProgress==0
    if (((I_k1>0)&&(Diff>0))||((I_k1<=0)&&(Diff<=0)))&&(abs(AxTarDt)<P_LongCtrl_VLCAxTarDtThreEnableI)
         t_I =Diff*tCycle;   
    else
         if abs(Diff)>P_LongCtrl_VLCcoefIFadeOut1Condition*Err
             t_I =P_LongCtrl_VLCcoefIFadeOut1Calc*Diff*tCycle;
         elseif abs(Diff)>P_LongCtrl_VLCcoefIFadeOut2Condition*Err
                 t_I =P_LongCtrl_VLCcoefIFadeOut2Calc*Diff*tCycle;
             elseif abs(Diff)>P_LongCtrl_VLCcoefIFadeOut3Condition*Err
                     t_I =P_LongCtrl_VLCcoefIFadeOut3Calc*Diff*tCycle;
                 else 
                     t_I =Diff*tCycle;
         end       
    end
    if ((abs(AxTarDt)<P_LongCtrl_VLCAxTarDtThreEnableI)&&(abs(Diff)<Err))
         if (abs(VlcAxTar)>0.001&&(abs(axvFilt)<Err))
             if VlcAxTar>0.001
                Icompension=P_LongCtrl_VLCIACompensionPos*tCycle;
             else
                if VlcAxTar<-0.001
                   Icompension=P_LongCtrl_VLCIACompensionNeg*tCycle;
                else
                   Icompension=single(0);
                end
             end
         else
             Icompension=single(0);
         end
         if (abs(VlcAxTar)<0.001&&(abs(axvFilt)<Err))
              Istability=-axvFilt*tCycle;
         else
             Istability=single(0);
         end         
    else
      Icompension=single(0);
      Istability=single(0);
    end   
          t_I=I_k1+t_I+Icompension+Istability; 
          t_I =max(min(P_VlcWindupLim,t_I),-P_VlcWindupLim);
          if (t_I==P_VlcWindupLim)||(t_I==(-P_VlcWindupLim))
              Limited =single(1);
          else
              Limited =single(0);
          end
          if ECenable  
             I = t_I;
          else
             I = single(0);
          end
else
      I = single(0.5)*I_k1;
      Limited=single(0);
end

== matlab function PvtSubSys_LONC/VLC/Vlc/SwitchToBrakeMode/Switch ==
  data: AxTarEnable input boolean; y output boolean; DevEnable input boolean; BrakePrefer input boolean; ACC_Mode input uint8; StopReq input boolean; Sw1 input boolean; Sw2 input boolean; Sw3 input boolean; Sw4 input boolean; Sw5 input boolean; Sw6 input boolean; Sw7 input boolean
function y = fcn(AxTarEnable,DevEnable,BrakePrefer,ACC_Mode,StopReq,Sw1,Sw2,Sw3,Sw4,Sw5,Sw6,Sw7)
%#codegen

if (ACC_Mode==6)||(ACC_Mode==9)||(StopReq==1)
   y=true;
else
   if BrakePrefer
       y = Sw1;
   else
      if (AxTarEnable==1)||(DevEnable==1)
          y = Sw1&&Sw2&&Sw3&&Sw4&&Sw7; 
      else
          y = Sw1&&Sw2&&Sw3&&Sw4&&Sw5&&Sw6&&Sw7; 
      end
   end
end

== matlab function PvtSubSys_LONC/VLC/Vlc/SwitchToDriveMode/Switch ==
  data: Active input; y output; BrakePrefer input; StopReq input; Sw1 input; Sw2 input; Sw3 input; Sw4 input; Sw5 input; DriveOff2EC input
function y = fcn(Active,BrakePrefer,StopReq,Sw1,Sw2,Sw3,Sw4,Sw5,DriveOff2EC)
%#codegen
if Active
   if BrakePrefer||StopReq
       y=false;
   else
      if Sw5
          y = Sw1;
      else
          y = Sw1&&Sw2&&Sw3&&Sw4;
      end
   end
   if DriveOff2EC
       y=true;
   end
else
    y=false;
end

== matlab function PvtSubSys_LONC/VLC/Vlc/UpdateFlagCalc/Timer/MATLAB Function ==
  data: Falling input; Timer output single; StartTimer output single; TimerK1 input; StartTimerK1 input
function [Timer,StartTimer]= fcn(Falling,TimerK1,StartTimerK1)
StartTimer=StartTimerK1;
Timer=single(0);
if Falling==1
    StartTimer=single(1);
end
if StartTimer==1
    Timer=TimerK1+single(0.02);
end
if Timer>0.5
    StartTimer=single(0);
end

== stateflow chart PvtSubSys_LONC/VLC/Vlc/VLC_control_sts ==
  settings: executeAtInitialization=1
  state Init
  state Failure
  state Off
  state Active
    state DC
      entry:DCEnable=true;
      entry:tDC=1;
      during:tDC=min(tDC+1,200);
      exit:DCEnable=false;
      exit:tDC=0;
    state EC
      entry:ECEnable=true;
      entry:tEC=1;
      during:tEC=min(tEC+1,200);
      exit:ECEnable=false;
      exit:tEC=0;
    state Override
    (junction 85) -> DC [order 1] : [(ACC_Mode==6)||(ACC_Mode==9)]
    (junction 85) -> EC [order 2] : [(ACC_Mode!=6)&&(ACC_Mode!=9)]
    EC -> DC [order 1] : [SwitchToBrakeMode==1]
    DC -> EC [order 1] : [(SwitchToDriveMode==1)&&(tDC>=25*Motorial)]
    (junction 60) -> DC [order 2] : [OverrideToDC==1]
    (junction 60) -> EC [order 1] : [OverrideToDC==0]
    Override -> (junction 60) : [ACC_Mode~=5]
    DC -> (junction 91) [order 2]
    EC -> (junction 91) [order 2]
    (junction 91) -> Override : [ACC_Mode==5]
  (default) -> Init
  Failure -> Init : [VLCInternalFailSts==0]
  Init -> (junction 30)
  (junction 30) -> Failure [order 1] : [VLCInternalFailSts==1]
  (junction 30) -> Off [order 2] : [VLCInternalFailSts==0]
  (junction 39) -> Failure : [VLCInternalFailSts==1]
  Off -> (junction 39) [order 2]
  Active -> (junction 39) [order 1]
  Off -> (junction 85) [order 1] : [(ACC_Mode==3)||...
      | (ACC_Mode==6)||...
      | (ACC_Mode==5)||...
      | (ACC_Mode==9)]
  Active -> Off [order 2] : [(ACC_Mode==0)||...
      | (ACC_Mode==1)||...
      | (ACC_Mode==2)||...
      | (ACC_Mode==7)]
  data: SwitchToDriveMode input; SwitchToBrakeMode input; ECEnable output boolean; tEC output single; tDC output single; ACC_Mode input; DCEnable output boolean; VLCInternalFailSts input; Motorial input single; OverrideToDC input single

== matlab function PvtSubSys_LONC/VLC/Vlc/VlcInternalAccCalc ==
  data: EC input; DC input; DriveOff input; ACC_Mode input; VlcInternalAcc output single; AxRef input; AxTar input; AcceJerk input; DeceJerk input; DriveOffAxUpLim input; VlcInternalAccK1 input
function VlcInternalAcc = CalcVlcInternalAcc(EC,DC,DriveOff,ACC_Mode,AxRef,AxTar,AcceJerk,DeceJerk,DriveOffAxUpLim,VlcInternalAccK1)
%#codegen
if ACC_Mode(1)==3
    if (DriveOff(1)==1)&&(DriveOff(2)==0)
           VlcInternalAcc = single(0.2);  
    else
       if ((VlcInternalAccK1>AxTar)&&(AxTar>=AxRef))||((VlcInternalAccK1<AxTar)&&(AxTar<=AxRef))
           VlcInternalAcc = AxTar;
       else
           if ((VlcInternalAccK1+DeceJerk*single(0.02))>AxRef)&&(AxRef>AxTar)
               VlcInternalAcc = AxRef+DeceJerk*single(0.02);
           else
               if ((VlcInternalAccK1+AcceJerk*single(0.02))<AxRef)&&(AxRef<AxTar)
                   VlcInternalAcc = AxRef+AcceJerk*single(0.02);
               else
                   VlcInternalAcc = max(min(AxTar,VlcInternalAccK1+AcceJerk*single(0.02)),VlcInternalAccK1+DeceJerk*single(0.02));
               end
           end
       end
    end
else
   if ACC_Mode(1)==6||ACC_Mode(1)==9
%        VlcInternalAcc=single(0);
       VlcInternalAcc = max(min(AxTar,VlcInternalAccK1+AcceJerk*single(0.02)),VlcInternalAccK1+DeceJerk*single(0.02));
   else
       VlcInternalAcc=AxRef;
   end
end
VlcInternalAcc = min(DriveOffAxUpLim,VlcInternalAcc);

== matlab function PvtSubSys_LONC/VLC/Vlc/Subsystem/MATLAB Function ==
  data: u input; ACCModeSts output; Counter input single; CounterK1 output single
function [ACCModeSts,CounterK1] = fcn(u,Counter)
if (u(1)==7)&&((u(2)==6)||u(2)==(9))
    Counter=single(76);
end
if Counter>0
    ACCModeSts=uint8(6);
    CounterK1=max(single(0),Counter-single(1));
else
    ACCModeSts = u(1);
    CounterK1=single(0);
end
